simulink model "power_brushlessDCmotor"  (R2020b)
settings: Solver=ode4  StartTime=0  StopTime=.2  FixedStep=Ts  MaxStep=1e-6  RelTol=1e-6  AbsTol=1e-6  EnableMultiTasking=on
PreLoadFcn:
  | assignin('base','Ts',[5e-6])
undefined symbols (not defined in the file or in its folder): Ts
libraries: powerlib x10, simulink x6, powerlib_meascontrol x3
Description:
  | This example illustrates use of the BLDC in a closed-loop
  | speed and voltage control on a 1 kW, 3000 rpm industrial motor
settings Model: ExtModeAutoUpdateStatusClock=off  Creator=MathWorks  LastModifiedBy=k
settings SolverCC: AutoScaleAbsTol=off
settings DataIOCC: LimitDataPoints=on  SaveFormat=Array  SignalLoggingSaveFormat=ModelDataLogs  ReturnWorkspaceOutputs=off  SignalLoggingName=sigsOut
settings OptimizationCC: ExpressionDepthLimit=2147483647  InitFltsAndDblsToZero=on  LifeSpan=inf
settings DebuggingCC: UnderspecifiedInitializationDetection=Classic  MergeDetectMultiDrivingBlocksExec=none  SignalResolutionControl=TryResolveAllWithWarning  MultiTaskDSMMsg=warning  MultiTaskCondExecSysMsg=none  FcnCallInpInsideContextMsg=warning  StateNameClashWarn=warning  SFUnexpectedBacktrackingDiag=warning  SFNoUnconditionalDefaultTransitionDiag=warning  SFExecutionAtInitializationDiag=none  ArithmeticOperatorsInVariantConditions=warning
settings HardwareCC: ProdBitPerPointer=32  ProdBitPerSizeT=32  ProdBitPerPtrDiffT=32  ProdLargestAtomicFloat=None  ProdIntDivRoundTo=Undefined  ProdEndianess=Unspecified  ProdWordSize=32  ProdHWDeviceType=32-bit Generic  TargetUnknown=on
settings ModelReferenceCC: PropagateSignalLabelsOutOfModel=off
settings SFSimCC: SimUseLocalCustomCode=off  CustomCodeUndefinedFunction=UseInterfaceOnly
settings RTWCC: RTWUseLocalCustomCode=off
settings CodeAppCC: StateflowObjectComments=on
settings GRTTargetCC: TargetLangStandard=C89/C90 (ANSI)  CombineOutputUpdateFcns=off  GRTInterface=on
settings ConfigComp: CovMetricSettings=dw  CovSaveCumulativeToWorkspaceVar=on  CovSaveSingleToWorkspaceVar=on  CovExternalEMLEnable=off  CovSFcnEnable=off
settings SimscapeCC: SimscapeNormalizeSystem=off

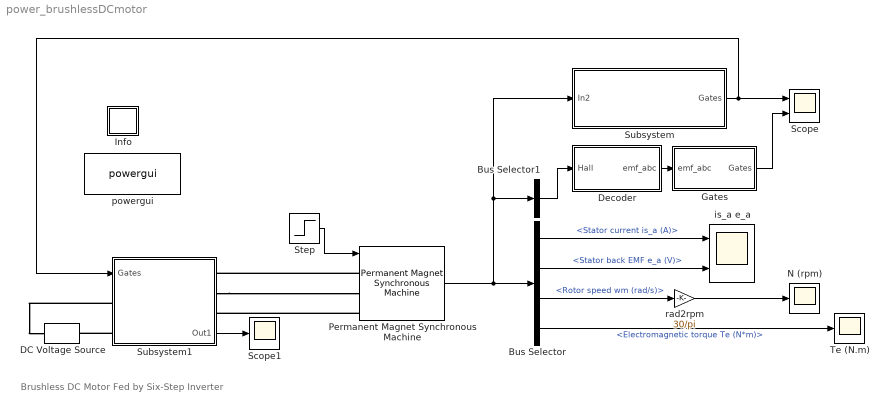
== system power_brushlessDCmotor ==
  note: Brushless DC Motor Fed by Six-Step Inverter
  Bus Selector : BusSelector  OutputSignals=Stator current is_a (A),Stator back EMF e_a (V),Rotor speed wm (rad/s),Electromagnetic torque Te (N*m)
  Bus Selector1 : BusSelector  OutputSignals=Hall effect signal h_a,Hall effect signal h_b,Hall effect signal h_c  OutputAsBus=on
  DC Voltage Source : powerlib/Electrical Sources/DC Voltage Source  Amplitude=200  Measurements=None
  Decoder : Subsystem
  Gates : Subsystem
  Info : Subsystem
      settings: OpenFcn=showdemo(bdroot(gcb))
      mask Display: disp('?')
  N (rpm) : Scope
  Permanent Magnet Synchronous Machine : powerlib/Machines/Permanent Magnet Synchronous Machine  NbPhases=3  FluxDistribution=Trapezoidal  RotorType=Round  MechanicalLoad=Torque Tm  PresetModel=No  ShowDetailedParameters=on  MeasurementBus=off  Resistance=2.8750  Inductance=8.5e-3  dqInductances=[8.5e-3, 8.5e-3]  La=0.000835  MachineConstant=Flux linkage established by magnets (V.s)  Flux=0.175  VoltageCst=146.6077  TorqueCst=1.4  Flat=120  Mechanical=[ 0.8e-3, 1e-3 4]  PolePairs=4  InitialConditions=[0,0, 0,0]  InitialConditions5ph=[0 0 0 0 0 0]  RefAngle=90 degrees behind phase A axis (modified Park)  IterativeDiscreteModel=Trapezoidal non iterative  TsBlock=-1  TsPowergui=0
  Scope : Scope  NumInputPorts=2
  Scope1 : Scope
  Step : Step  Time=.1  After=3  SampleTime=0
  Subsystem : Subsystem
  Subsystem1 : Subsystem
      settings: PortSchema="{\"entries\":[{\"content\":{\"sides\":[{\"content\":{\"connectorIds\":[\"In1\",\"LConn1\",\"LConn2\"]},\"type\":\"ConnectorPlacement.EquallySpacedRectSide\",\"uuid\":\"3e830c6c-b48e-4079-a555-63399f867b77\"},{\"content\":{\"connectorIds\":[\"RConn1\",\"RConn2\",\"RConn3\",\"Out1\"],\"side\":\"RIGHT\"},\"type\":\"ConnectorPlacement.EquallySpacedRectSide\",\"uuid\":\"e14bd0c3-2e36-4f0a-b270-beb41da57375\"},{\"content\":{\"connectorIds\":[],\"side\":\"TOP\"},\"type\":\"ConnectorPlacement.EquallySpacedRectSide\",\"uuid\":\"09179360-9fc0-4e49-92b5-7039012dd2c1\"},{\"content\":{\"connectorIds\":[],\"side\":\"HIDDEN\"},\"type\":\"ConnectorPlacement.EquallySpacedRectSide\",\"uuid\":\"af73253b-f07c-4a33-82ef-931e630f0fb0\"}]},\"type\":\"ConnectorPlacement.EquallySpacedConnector\",\"uuid\":\"7ce09c9c-6d00-4ec6-ad58-4c4a30439337\"}],\"packageUris\":[\"http://schema.mathworks.com/mf0/Connector/R2020b\"],\"version\":\"1.0\"}"
  Te (N.m) : Scope
  is_a e_a : Scope  NumInputPorts=2
  powergui : powerlib/powergui  Priority=2  SimulationMode=Discrete  SampleTime=Ts  frequency=60  Iterations=50  frequencyindice=0  Pbase=100e6  ErrMax=1e-4  UnitsV=kV  UnitsW=MW  buscounter=0  FunctionMessages=off  echomessages=off  EnableUseOfTLC=off  CurrentSourceSwitches=off  DisableSnubberDevices=off  DisableRonSwitches=off  DisableVfSwitches=off  DisplayEquations=off  AutomaticDiscreteSolvers=off  SolverType=Tustin/Backward Euler (TBE)  Interpol=off  ExternalGateDelay=off  methode=off  Ts=0  x0status=blocks  SPID=off  SwTol=0  HookPort=off  NonlinearTolerance=1e-4  nMaxIteration=100  ContinueOnMaxIteration=off  RestoreLinks=warning  ResistiveCurrentMeasurement=off  Frange=[0:2:500]  Ylog=off  Xlog=on  ShowGrid=off  save=off  variable=ZData  structure=0  ZoomFFT=on  StartTime=0.0  cycles=1  DisplayStyle=1  fundamental=60  FreqAxis=off  MaxFrequency=1000  frequencyindicesteady=1  RmsSteady=1  display=off
  rad2rpm : Gain  Gain=30/pi
  wires:
  Step/1 -> Permanent Magnet Synchronous Machine/1
  Gates/1(Gates) -> Scope/2
  Decoder/1(emf_abc) -> Gates/1("emf_abc ")
  rad2rpm/1 -> N (rpm)/1
  Bus Selector/1 -> is_a e_a/1  "<Stator current is_a (A)>"
  Permanent Magnet Synchronous Machine/1 -> Bus Selector1/1, Subsystem/1(In2), Bus Selector/1
  Bus Selector/2 -> is_a e_a/2  "<Stator back EMF e_a (V)>"
  Bus Selector/3 -> rad2rpm/1  "<Rotor speed wm (rad/s)>"
  Bus Selector/4 -> Te (N.m)/1  "<Electromagnetic torque Te (N*m)>"
  Bus Selector1/1 -> Decoder/1("Hall ")
  Subsystem/1(Gates) -> Subsystem1/1(Gates), Scope/1
  Subsystem1/1(Out1) -> Scope1/1
  connections:
  Permanent Magnet Synchronous Machine/LConn1 -- Subsystem1/RConn1
  Subsystem1/RConn2 -- Permanent Magnet Synchronous Machine/LConn2
  Permanent Magnet Synchronous Machine/LConn3 -- Subsystem1/RConn3
  Subsystem1/LConn1 -- DC Voltage Source/RConn1
  Subsystem1/LConn2 -- DC Voltage Source/LConn1

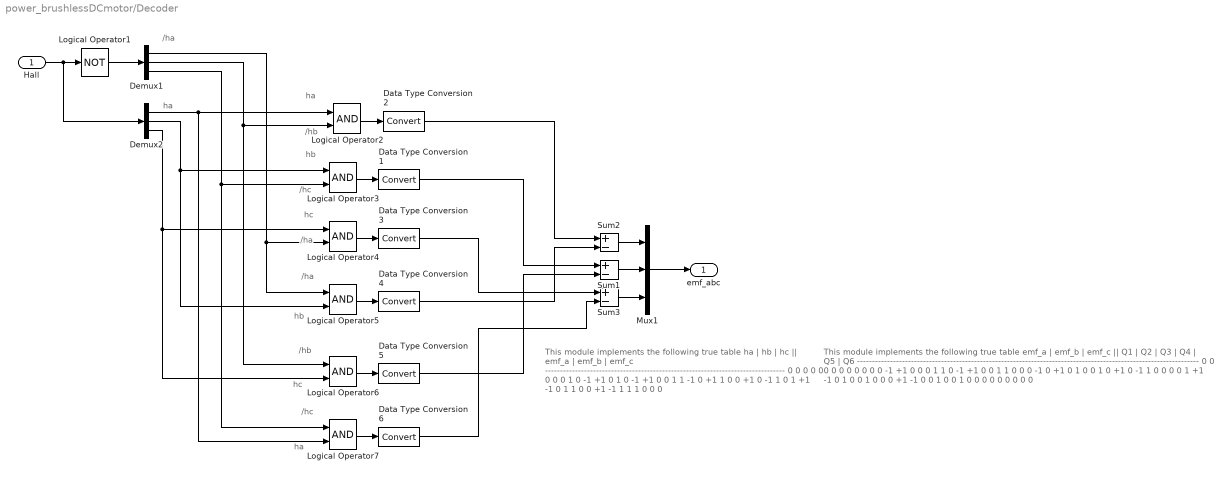
== system power_brushlessDCmotor/Decoder ==
  note: /ha
  note: ha
  note: ha
  note: /hb
  note: hb
  note: /hc
  note: hc
  note: /ha
  note: /ha
  note: hb
  note: /hb
  note: hc
  note: /hc
  note: ha
  note: This module implements the following true table
      |
      |    ha   |   hb   |   hc   ||   emf_a   |   emf_b   |   emf_c
      |     --------------------------------------------------------------------------------
      | 0          0         0          0               0               0
      | 0          0         1          0               -1              +1
      | 0          1         0          -1              +1                0
      | 0          1         1          -1               0               +1
      | 1          0         0         +1               0               -1
      | 1          0         1         +1              -1                0
      | 1          1         0          0              +1               -1
      | 1          1         1          0               0                0
  note: This module implements the following true table
      |
      |    emf_a   |   emf_b   |   emf_c   ||   Q1   |   Q2   |   Q3   |   Q4   |   Q5   |   Q6
      |     ------------------------------------------------------------------------------------------------------------------
      |       0              0                0            0          0          0           0        0        0
      |       0               -1              +1          0          0          0           1        1        0
      |     -1              +1                0          0          1          1           0        0        0
      |     -1               0               +1          0          1         0           0        1        0
      |    +1               0                -1          1          0          0           0        0        1
      |    +1              -1                0           1          0          0           1        0        0
      |      0              +1               -1           0          0          1           0        0        1
      |     0              0                0             0          0          0           0        0        0
  "Hall " : Inport
  Data Type Conversion{1..6} (6 alike) : DataTypeConversion
  Demux1 : Demux  Outputs=3
  Demux2 : Demux  Outputs=3
  Logical Operator1 : Logic  Operator=NOT  AllPortsSameDT=off  OutDataTypeStr=boolean
  Logical Operator{2..7} (6 alike) : Logic  AllPortsSameDT=off  OutDataTypeStr=boolean
  Mux1 : Mux  Inputs=3
  Sum1 : Sum  Inputs=+-  OutDataTypeStr=double
  Sum2 : Sum  Inputs=+-  OutDataTypeStr=double
  Sum3 : Sum  Inputs=+-  OutDataTypeStr=double
  emf_abc : Outport  VectorParamsAs1DForOutWhenUnconnected=off
  wires:
  "Hall "/1 -> Logical Operator1/1, Demux2/1
  Logical Operator1/1 -> Demux1/1
  Demux2/3 -> Logical Operator4/1, Logical Operator6/2
  Demux2/2 -> Logical Operator3/1, Logical Operator5/2
  Demux2/1 -> Logical Operator2/1, Logical Operator7/2
  Demux1/3 -> Logical Operator3/2, Logical Operator7/1
  Demux1/2 -> Logical Operator2/2, Logical Operator6/1
  Demux1/1 -> Logical Operator4/2, Logical Operator5/1
  Logical Operator2/1 -> Data Type Conversion2/1
  Sum2/1 -> Mux1/1
  Sum1/1 -> Mux1/2
  Sum3/1 -> Mux1/3
  Mux1/1 -> emf_abc/1
  Logical Operator3/1 -> Data Type Conversion1/1
  Logical Operator4/1 -> Data Type Conversion3/1
  Logical Operator5/1 -> Data Type Conversion4/1
  Logical Operator6/1 -> Data Type Conversion5/1
  Logical Operator7/1 -> Data Type Conversion6/1
  Data Type Conversion2/1 -> Sum2/1
  Data Type Conversion4/1 -> Sum2/2
  Data Type Conversion1/1 -> Sum1/1
  Data Type Conversion5/1 -> Sum1/2
  Data Type Conversion3/1 -> Sum3/1
  Data Type Conversion6/1 -> Sum3/2

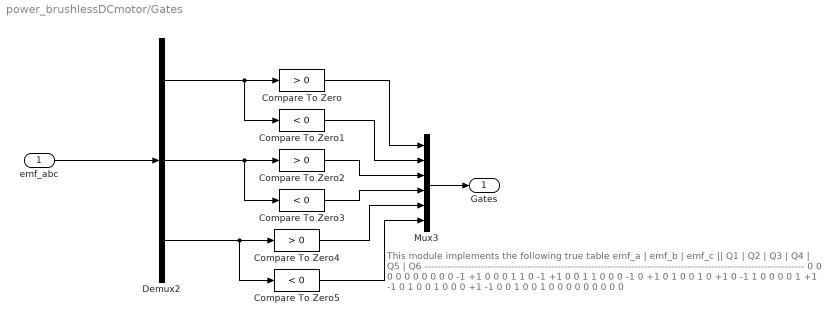
== system power_brushlessDCmotor/Gates ==
  note: This module implements the following true table
      |
      |    emf_a   |   emf_b   |   emf_c   ||   Q1   |   Q2   |   Q3   |   Q4   |   Q5   |   Q6
      |     ------------------------------------------------------------------------------------------------------------------
      |       0              0                0            0          0          0           0        0        0
      |       0               -1              +1          0          0          0           1        1        0
      |     -1              +1                0          0          1          1           0        0        0
      |     -1               0               +1          0          1         0           0        1        0
      |    +1               0                -1          1          0          0           0        0        1
      |    +1              -1                0           1          0          0           1        0        0
      |      0              +1               -1           0          0          1           0        0        1
      |     0              0                0             0          0          0           0        0        0
  "emf_abc " : Inport
  Compare To Zero : simulink/Logic and Bit Operations/Compare To Zero  relop=>  OutDataTypeStr=boolean  ZeroCross=off
  Compare To Zero1 : simulink/Logic and Bit Operations/Compare To Zero  relop=<  OutDataTypeStr=boolean  ZeroCross=off
  Compare To Zero2 : simulink/Logic and Bit Operations/Compare To Zero  relop=>  OutDataTypeStr=boolean  ZeroCross=off
  Compare To Zero3 : simulink/Logic and Bit Operations/Compare To Zero  relop=<  OutDataTypeStr=boolean  ZeroCross=off
  Compare To Zero4 : simulink/Logic and Bit Operations/Compare To Zero  relop=>  OutDataTypeStr=boolean  ZeroCross=off
  Compare To Zero5 : simulink/Logic and Bit Operations/Compare To Zero  relop=<  OutDataTypeStr=boolean  ZeroCross=off
  Demux2 : Demux  Outputs=3
  Mux3 : Mux  Inputs=6
  Gates : Outport  VectorParamsAs1DForOutWhenUnconnected=off
  wires:
  "emf_abc "/1 -> Demux2/1
  Mux3/1 -> Gates/1
  Demux2/1 -> Compare To Zero/1, Compare To Zero1/1
  Demux2/2 -> Compare To Zero2/1, Compare To Zero3/1
  Demux2/3 -> Compare To Zero4/1, Compare To Zero5/1
  Compare To Zero/1 -> Mux3/1
  Compare To Zero1/1 -> Mux3/2
  Compare To Zero2/1 -> Mux3/3
  Compare To Zero3/1 -> Mux3/4
  Compare To Zero4/1 -> Mux3/5
  Compare To Zero5/1 -> Mux3/6

== system power_brushlessDCmotor/Info ==

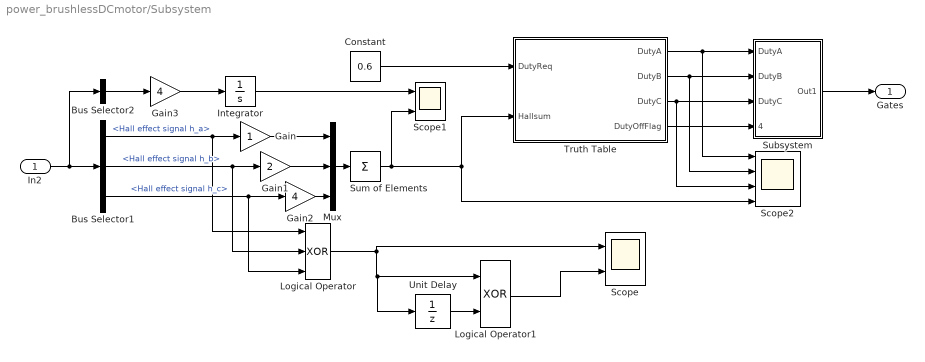
== system power_brushlessDCmotor/Subsystem ==
  In2 : Inport
  Bus Selector1 : BusSelector  OutputSignals=Hall effect signal h_a,Hall effect signal h_b,Hall effect signal h_c
  Bus Selector2 : BusSelector  OutputSignals=Rotor speed wm (rad/s)  OutputAsBus=on
  Constant : Constant  Value=0.6
  Gain : Gain
  Gain1 : Gain  Gain=2
  Gain2 : Gain  Gain=4
  Gain3 : Gain  Gain=4
  Integrator : Integrator  WrapState=on
  Logical Operator : Logic  Operator=XOR  Inputs=3  AllPortsSameDT=off  OutDataTypeStr=boolean
  Logical Operator1 : Logic  Operator=XOR  AllPortsSameDT=off  OutDataTypeStr=boolean
  Mux : Mux  Inputs=3
  Scope : Scope  NumInputPorts=2
  Scope1 : Scope  NumInputPorts=2
  Scope2 : Scope  NumInputPorts=4
  Subsystem : Subsystem
  Sum of Elements : Sum  Inputs=+
  Truth Table : Truth Table  TreatAsAtomicUnit=on
      settings: PortSchema="{\"entries\":[{\"content\":{\"sides\":[{\"content\":{\"connectorIds\":[\"In2\",\"In1\"]},\"type\":\"ConnectorPlacement.EquallySpacedRectSide\",\"uuid\":\"59c0d94d-4ab6-4082-9c20-9efdae7878b3\"},{\"content\":{\"connectorIds\":[\"Out1\",\"Out2\",\"Out3\",\"Out4\"],\"side\":\"RIGHT\"},\"type\":\"ConnectorPlacement.EquallySpacedRectSide\",\"uuid\":\"fbebaf7f-5920-4df9-84a7-9b0467c91c72\"},{\"content\":{\"connectorIds\":[],\"side\":\"TOP\"},\"type\":\"ConnectorPlacement.EquallySpacedRectSide\",\"uuid\":\"8ff1c87b-d4dc-46a0-9459-25a6278b9f20\"},{\"content\":{\"connectorIds\":[],\"side\":\"HIDDEN\"},\"type\":\"ConnectorPlacement.EquallySpacedRectSide\",\"uuid\":\"16bdd2e1-f1a8-43ed-aa1c-d33053eb9e05\"}]},\"type\":\"ConnectorPlacement.EquallySpacedConnector\",\"uuid\":\"7896656f-e18e-44d5-80e3-9050e65d4579\"}],\"packageUris\":[\"http://schema.mathworks.com/mf0/Connector/R2020b\"],\"version\":\"1.0\"}"
  Unit Delay : UnitDelay  SampleTime=-1  HasFrameUpgradeWarning=on
  Gates : Outport
  wires:
  Gain1/1 -> Mux/2
  Logical Operator1/1 -> Scope/2
  Bus Selector1/1 -> Gain/1, Logical Operator/1  "<Hall effect signal h_a>"
  Unit Delay/1 -> Logical Operator1/2
  Sum of Elements/1 -> Truth Table/1(Hallsum), Scope2/4, Scope1/2
  Bus Selector1/3 -> Gain2/1, Logical Operator/3  "<Hall effect signal h_c>"
  Gain2/1 -> Mux/3
  Bus Selector2/1 -> Gain3/1
  Mux/1 -> Sum of Elements/1
  Integrator/1 -> Scope1/1
  Logical Operator/1 -> Unit Delay/1, Logical Operator1/1, Scope/1
  Gain/1 -> Mux/1
  Truth Table/1(DutyA) -> Subsystem/1(DutyA), Scope2/1
  Gain3/1 -> Integrator/1
  Truth Table/3(DutyC) -> Scope2/3, Subsystem/3(DutyC)
  Truth Table/2(DutyB) -> Scope2/2, Subsystem/2(DutyB)
  Constant/1 -> Truth Table/2(DutyReq)
  In2/1 -> Bus Selector2/1, Bus Selector1/1
  Bus Selector1/2 -> Gain1/1, Logical Operator/2  "<Hall effect signal h_b>"
  Subsystem/1(Out1) -> Gates/1
  Truth Table/4(DutyOffFlag) -> Subsystem/4(DutyOffFlag)

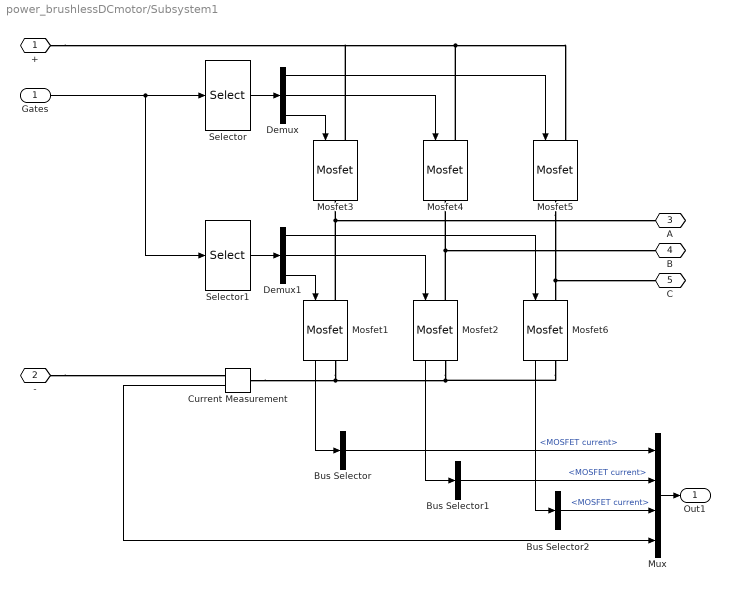
== system power_brushlessDCmotor/Subsystem1 ==
  Gates : Inport
  Bus Selector : BusSelector  OutputSignals=MOSFET current
  Bus Selector1 : BusSelector  OutputSignals=MOSFET current
  Bus Selector2 : BusSelector  OutputSignals=MOSFET current
  Current Measurement : powerlib/Measurements/Current Measurement  PhasorSimulation=off  OutputType=Complex  PSBequivalent=0
  Demux : Demux  Outputs=3
  Demux1 : Demux  Outputs=3
  Mosfet1 : powerlib/Power Electronics/Mosfet  Ron=0.001  Lon=0  Rd=0.0001  Vfd=0  IC=0  Rs=1e5  Cs=inf  Measurements=on
  Mosfet2 : powerlib/Power Electronics/Mosfet  Ron=0.001  Lon=0  Rd=0.0001  Vfd=0  IC=0  Rs=1e5  Cs=inf  Measurements=on
  Mosfet3 : powerlib/Power Electronics/Mosfet  Ron=0.001  Lon=0  Rd=0.0001  Vfd=0  IC=0  Rs=1e5  Cs=inf  Measurements=off
  Mosfet4 : powerlib/Power Electronics/Mosfet  Ron=0.001  Lon=0  Rd=0.0001  Vfd=0  IC=0  Rs=1e5  Cs=inf  Measurements=off
  Mosfet5 : powerlib/Power Electronics/Mosfet  Ron=0.001  Lon=0  Rd=0.0001  Vfd=0  IC=0  Rs=1e5  Cs=inf  Measurements=off
  Mosfet6 : powerlib/Power Electronics/Mosfet  Ron=0.001  Lon=0  Rd=0.0001  Vfd=0  IC=0  Rs=1e5  Cs=inf  Measurements=on
  Mux : Mux
  Selector : Selector  InputPortWidth=6  IndexOptions=Index vector (dialog)  Indices=[5 3 1]  OutputSizes=1
  Selector1 : Selector  InputPortWidth=6  IndexOptions=Index vector (dialog)  Indices=[6 4 2]  OutputSizes=1
  + : PMIOPort  Side=Left
  - : PMIOPort  Port=2  Side=Left
  A : PMIOPort  Port=3  Side=Right
  B : PMIOPort  Port=4  Side=Right
  C : PMIOPort  Port=5  Side=Right
  Out1 : Outport
  wires:
  Bus Selector1/1 -> Mux/2  "<MOSFET current>"
  Bus Selector2/1 -> Mux/3  "<MOSFET current>"
  Bus Selector/1 -> Mux/1  "<MOSFET current>"
  Mosfet1/1 -> Bus Selector/1
  Mosfet6/1 -> Bus Selector2/1
  Mosfet2/1 -> Bus Selector1/1
  Selector/1 -> Demux/1
  Gates/1 -> Selector1/1, Selector/1
  Current Measurement/1 -> Mux/4
  Mux/1 -> Out1/1
  Demux/1 -> Mosfet5/1
  Demux/2 -> Mosfet4/1
  Demux/3 -> Mosfet3/1
  Selector1/1 -> Demux1/1
  Demux1/3 -> Mosfet1/1
  Demux1/2 -> Mosfet2/1
  Demux1/1 -> Mosfet6/1
  connections:
  Mosfet2/LConn1 -- Mosfet4/RConn1 -- B/RConn1
  Mosfet1/RConn1 -- Mosfet6/RConn1 -- Mosfet2/RConn1 -- Current Measurement/LConn1
  Mosfet4/LConn1 -- Mosfet5/LConn1 -- Mosfet3/LConn1 -- +/RConn1
  Mosfet5/RConn1 -- Mosfet6/LConn1 -- C/RConn1
  Mosfet1/LConn1 -- A/RConn1 -- Mosfet3/RConn1
  -/RConn1 -- Current Measurement/RConn1

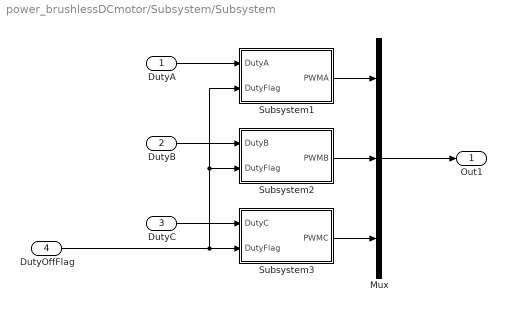
== system power_brushlessDCmotor/Subsystem/Subsystem ==
  DutyA : Inport
  DutyB : Inport  Port=2
  DutyC : Inport  Port=3
  DutyOffFlag : Inport  Port=4
  Mux : Mux  Inputs=3
  Subsystem1 : Subsystem
  Subsystem2 : Subsystem
  Subsystem3 : Subsystem
  Out1 : Outport
  wires:
  Mux/1 -> Out1/1
  Subsystem1/1(PWMA) -> Mux/1
  DutyA/1 -> Subsystem1/1(DutyA)
  Subsystem2/1(PWMB) -> Mux/2
  Subsystem3/1(PWMC) -> Mux/3
  DutyB/1 -> Subsystem2/1(DutyB)
  DutyC/1 -> Subsystem3/1(DutyC)
  DutyOffFlag/1 -> Subsystem1/2(DutyFlag), Subsystem2/2(DutyFlag), Subsystem3/2(DutyFlag)

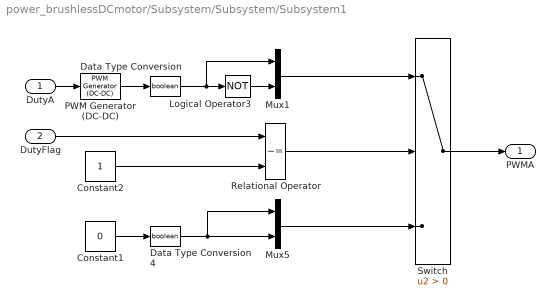
== system power_brushlessDCmotor/Subsystem/Subsystem/Subsystem1 ==
  DutyA : Inport
  DutyFlag : Inport  Port=2
  Constant1 : Constant  Value=0
  Constant2 : Constant
  Data Type Conversion : DataTypeConversion  OutDataTypeStr=boolean
  Data Type Conversion4 : DataTypeConversion  OutDataTypeStr=boolean
  Logical Operator3 : Logic  Operator=NOT  AllPortsSameDT=off  OutDataTypeStr=boolean
  Mux1 : Mux  Inputs=2
  Mux5 : Mux  Inputs=2
  PWM Generator (DC-DC) : powerlib_meascontrol/Pulse & Signal Generators/PWM Generator (DC-DC)  Fsw=10000  Ts=5e-6
  Relational Operator : RelationalOperator  Operator=~=  OutDataTypeStr=boolean  RndMeth=Simplest
  Switch : Switch  Criteria=u2 > Threshold
  PWMA : Outport
  wires:
  Data Type Conversion/1 -> Logical Operator3/1, Mux1/1
  Mux1/1 -> Switch/1
  DutyA/1 -> PWM Generator (DC-DC)/1
  Mux5/1 -> Switch/3
  PWM Generator (DC-DC)/1 -> Data Type Conversion/1
  Constant1/1 -> Data Type Conversion4/1
  Logical Operator3/1 -> Mux1/2
  Data Type Conversion4/1 -> Mux5/2, Mux5/1
  Constant2/1 -> Relational Operator/2
  DutyFlag/1 -> Relational Operator/1
  Switch/1 -> PWMA/1
  Relational Operator/1 -> Switch/2

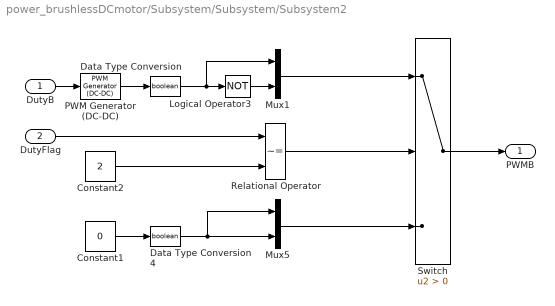
== system power_brushlessDCmotor/Subsystem/Subsystem/Subsystem2 ==
  DutyB : Inport
  DutyFlag : Inport  Port=2
  Constant1 : Constant  Value=0
  Constant2 : Constant  Value=2
  Data Type Conversion : DataTypeConversion  OutDataTypeStr=boolean
  Data Type Conversion4 : DataTypeConversion  OutDataTypeStr=boolean
  Logical Operator3 : Logic  Operator=NOT  AllPortsSameDT=off  OutDataTypeStr=boolean
  Mux1 : Mux  Inputs=2
  Mux5 : Mux  Inputs=2
  PWM Generator (DC-DC) : powerlib_meascontrol/Pulse & Signal Generators/PWM Generator (DC-DC)  Fsw=10000  Ts=5e-6
  Relational Operator : RelationalOperator  Operator=~=  OutDataTypeStr=boolean  RndMeth=Simplest
  Switch : Switch  Criteria=u2 > Threshold
  PWMB : Outport
  wires:
  Relational Operator/1 -> Switch/2
  Switch/1 -> PWMB/1
  DutyFlag/1 -> Relational Operator/1
  Constant2/1 -> Relational Operator/2
  Data Type Conversion4/1 -> Mux5/1, Mux5/2
  Logical Operator3/1 -> Mux1/2
  Constant1/1 -> Data Type Conversion4/1
  PWM Generator (DC-DC)/1 -> Data Type Conversion/1
  Mux5/1 -> Switch/3
  DutyB/1 -> PWM Generator (DC-DC)/1
  Mux1/1 -> Switch/1
  Data Type Conversion/1 -> Mux1/1, Logical Operator3/1

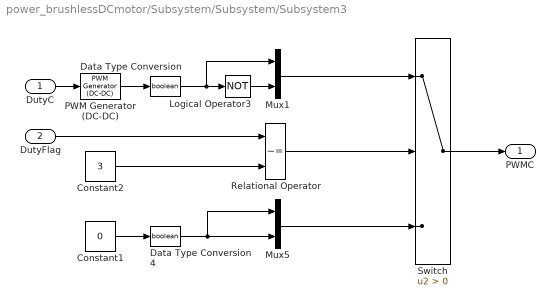
== system power_brushlessDCmotor/Subsystem/Subsystem/Subsystem3 ==
  DutyC : Inport
  DutyFlag : Inport  Port=2
  Constant1 : Constant  Value=0
  Constant2 : Constant  Value=3
  Data Type Conversion : DataTypeConversion  OutDataTypeStr=boolean
  Data Type Conversion4 : DataTypeConversion  OutDataTypeStr=boolean
  Logical Operator3 : Logic  Operator=NOT  AllPortsSameDT=off  OutDataTypeStr=boolean
  Mux1 : Mux  Inputs=2
  Mux5 : Mux  Inputs=2
  PWM Generator (DC-DC) : powerlib_meascontrol/Pulse & Signal Generators/PWM Generator (DC-DC)  Fsw=10000  Ts=5e-6
  Relational Operator : RelationalOperator  Operator=~=  OutDataTypeStr=boolean  RndMeth=Simplest
  Switch : Switch  Criteria=u2 > Threshold
  PWMC : Outport
  wires:
  Data Type Conversion/1 -> Logical Operator3/1, Mux1/1
  Mux1/1 -> Switch/1
  DutyC/1 -> PWM Generator (DC-DC)/1
  Mux5/1 -> Switch/3
  PWM Generator (DC-DC)/1 -> Data Type Conversion/1
  Constant1/1 -> Data Type Conversion4/1
  Logical Operator3/1 -> Mux1/2
  Data Type Conversion4/1 -> Mux5/2, Mux5/1
  Constant2/1 -> Relational Operator/2
  DutyFlag/1 -> Relational Operator/1
  Switch/1 -> PWMC/1
  Relational Operator/1 -> Switch/2

== matlab function power_brushlessDCmotor/Subsystem/Truth Table ==
  data: Hallsum input; DutyA output; DutyB output; DutyC output; DutyReq input; DutyOffFlag output double
function [DutyA, DutyB, DutyC, DutyOffFlag] = fcn(Hallsum, DutyReq)

aVarTruthTableCondition_1 = false;
aVarTruthTableCondition_2 = false;
aVarTruthTableCondition_3 = false;
aVarTruthTableCondition_4 = false;
aVarTruthTableCondition_5 = false;
aVarTruthTableCondition_6 = false;


% Condition #1
aVarTruthTableCondition_1 = logical(Hallsum == 1);

% Condition #2
aVarTruthTableCondition_2 = logical(Hallsum == 2);

% Condition #3
aVarTruthTableCondition_3 = logical(Hallsum == 3);

% Condition #4
aVarTruthTableCondition_4 = logical(Hallsum == 4);

% Condition #5
aVarTruthTableCondition_5 = logical(Hallsum == 5);

% Condition #6
aVarTruthTableCondition_6 = logical(Hallsum == 6);

if (aVarTruthTableCondition_1 && ~aVarTruthTableCondition_2 && ~aVarTruthTableCondition_3 && ~aVarTruthTableCondition_4 && ~aVarTruthTableCondition_5 && ~aVarTruthTableCondition_6)
    aFcnTruthTableAction_1();
elseif (~aVarTruthTableCondition_1 && aVarTruthTableCondition_2 && ~aVarTruthTableCondition_3 && ~aVarTruthTableCondition_4 && ~aVarTruthTableCondition_5 && ~aVarTruthTableCondition_6)
    aFcnTruthTableAction_2();
elseif (~aVarTruthTableCondition_1 && ~aVarTruthTableCondition_2 && aVarTruthTableCondition_3 && ~aVarTruthTableCondition_4 && ~aVarTruthTableCondition_5 && ~aVarTruthTableCondition_6)
    aFcnTruthTableAction_3();
elseif (~aVarTruthTableCondition_1 && ~aVarTruthTableCondition_2 && ~aVarTruthTableCondition_3 && aVarTruthTableCondition_4 && ~aVarTruthTableCondition_5 && ~aVarTruthTableCondition_6)
    aFcnTruthTableAction_4();
elseif (~aVarTruthTableCondition_1 && ~aVarTruthTableCondition_2 && ~aVarTruthTableCondition_3 && ~aVarTruthTableCondition_4 && aVarTruthTableCondition_5 && ~aVarTruthTableCondition_6)
    aFcnTruthTableAction_5();
elseif (~aVarTruthTableCondition_1 && ~aVarTruthTableCondition_2 && ~aVarTruthTableCondition_3 && ~aVarTruthTableCondition_4 && ~aVarTruthTableCondition_5 && aVarTruthTableCondition_6)
    aFcnTruthTableAction_6();
else % Default
    aFcnTruthTableAction_7();
end

function aFcnTruthTableAction_1()

% Example action 1 called from D1 & D2 column in condition table

DutyA = DutyReq;
DutyB = 0;
DutyC = 0;
DutyOffFlag = 2;

function aFcnTruthTableAction_2()

% Example action 2 called from D3 column in condition table

DutyA = 0;
DutyB = DutyReq;
DutyC = 0;
DutyOffFlag = 3;

function aFcnTruthTableAction_3()



DutyA = 0;
DutyB = DutyReq;
DutyC = 0;
DutyOffFlag = 1;

function aFcnTruthTableAction_4()



DutyA = 0;
DutyB = 0;
DutyC = DutyReq;
DutyOffFlag = 1;

function aFcnTruthTableAction_5()



DutyA = DutyReq;
DutyB = 0;
DutyC = 0;
DutyOffFlag = 3;

function aFcnTruthTableAction_6()



DutyA = 0;
DutyB = 0;
DutyC = DutyReq;
DutyOffFlag = 2;

function aFcnTruthTableAction_7()



DutyA = 0;
DutyB = 0;
DutyC = 0;
DutyOffFlag = 0;
